simulink model "carSim"  (R2020a)
settings: Solver=FixedStepAuto  StartTime=0.0  StopTime=150  FixedStep=0.1406  MaxStep=0.1  RelTol=1e-3
model workspace: external: MATLAB File C:\Users\chsl\Documents\teaching\Reguleringsteknik (4. semester)\matlab\handInExercises\ex2Init.m (data not in the file)
values from neighbouring files (symbols this model uses):
  c = 10    [ex2Init.m]
  g = 9.82    [ex2Init.m]
  m = 900    [ex2Init.m]
  vBar = 10    [ex2Init.m]
settings Model: Creator=chsl  LastModifiedBy=madsw
settings DataIOCC: ReturnWorkspaceOutputs=off
settings DebuggingCC: ArithmeticOperatorsInVariantConditions=warning
settings SFSimCC: SimUseLocalCustomCode=off  CustomCodeUndefinedFunction=UseInterfaceOnly
settings RTWCC: RTWUseLocalCustomCode=off

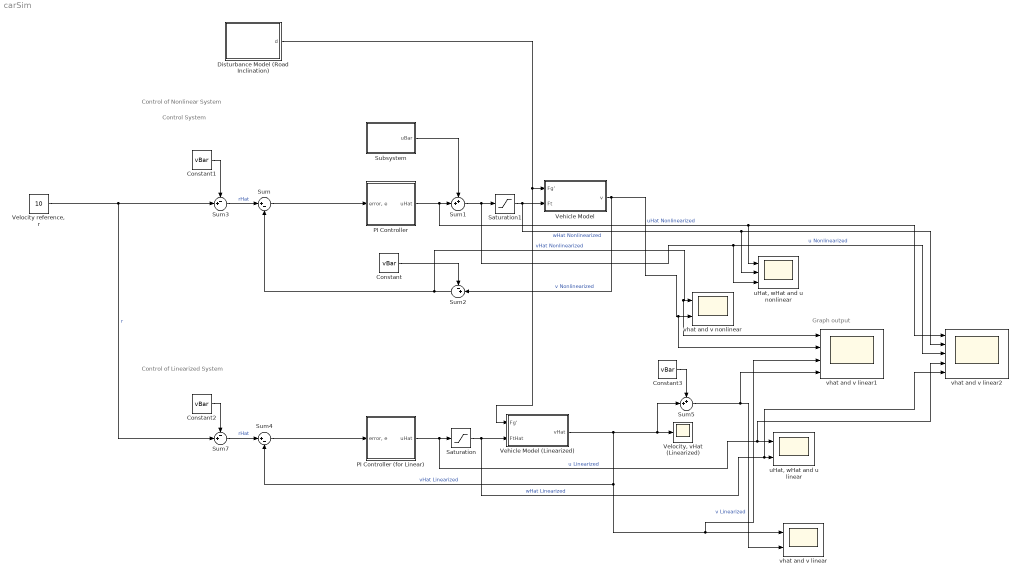
== system carSim ==
  note: Graph output
  note: Control System
  note: Control of Nonlinear System
  note: Control of Linearized System
  Constant{,1..3} (4 alike) : Constant  Value=vBar
  "Disturbance Model (Road Inclination) " : Subsystem
  PI Controller : Subsystem
  PI Controller (for Linear) : Subsystem
  Saturation : Saturate  UpperLimit=3000  LowerLimit=-3000
  Saturation1 : Saturate  UpperLimit=3000  LowerLimit=-3000
  Subsystem : Subsystem
  Sum : Sum  Inputs=|+-
  Sum1 : Sum  Inputs=++|
  Sum2 : Sum  Inputs=-+|
  Sum3 : Sum  Inputs=-+|
  Sum4 : Sum  Inputs=|+-
  Sum5 : Sum  Inputs=++|
  Sum7 : Sum  Inputs=-+|
  Vehicle Model : Subsystem
  Vehicle Model (Linearized) : Subsystem
  "Velocity reference, r" : Constant  Value=10
  "Velocity, vHat (Linearized)" : Scope
  "uHat, wHat and u linear" : Scope  NumInputPorts=2
  "uHat, wHat and u nonlinear" : Scope  NumInputPorts=3
  vhat and v linear : Scope  NumInputPorts=2
  vhat and v linear1 : Scope  NumInputPorts=4
  vhat and v linear2 : Scope  NumInputPorts=5
  vhat and v nonlinear : Scope  NumInputPorts=2
  wires:
  "Disturbance Model (Road Inclination) "/1(d) -> Vehicle Model (Linearized)/1(Fg'), Vehicle Model/1(Fg')
  Sum/1 -> PI Controller/1("error, e")
  Sum1/1 -> Saturation1/1, vhat and v linear2/3, "uHat, wHat and u nonlinear"/3  "u Nonlinearized"
  PI Controller/1(uHat) -> "uHat, wHat and u nonlinear"/1, vhat and v linear2/1, Sum1/2  "uHat Nonlinearized"
  Subsystem/1(uBar) -> Sum1/1
  Constant/1 -> Sum2/1
  Vehicle Model/1(v) -> Sum2/2, vhat and v linear1/2, vhat and v nonlinear/2  "v Nonlinearized"
  Sum2/1 -> vhat and v linear1/1, vhat and v nonlinear/1, Sum/2  "vHat Nonlinearized"
  Constant1/1 -> Sum3/1
  Sum4/1 -> PI Controller (for Linear)/1("error, e")
  Sum3/1 -> Sum/1  "rHat"
  PI Controller (for Linear)/1(uHat) -> vhat and v linear2/4, "uHat, wHat and u linear"/1, Saturation/1  "u Linearized"
  Constant2/1 -> Sum7/1
  "Velocity reference, r"/1 -> Sum7/2, Sum3/2  "r"
  Sum7/1 -> Sum4/1  "rHat"
  Constant3/1 -> Sum5/1
  Sum5/1 -> vhat and v linear/2, vhat and v linear1/4  "v Linearized"
  Saturation1/1 -> Vehicle Model/2(Ft), vhat and v linear2/2, "uHat, wHat and u nonlinear"/2  "wHat Nonlinearized"
  Vehicle Model (Linearized)/1(vHat) -> vhat and v linear1/3, vhat and v linear/1, Sum4/2, Sum5/2, "Velocity, vHat (Linearized)"/1  "vHat Linearized"
  Saturation/1 -> vhat and v linear2/5, "uHat, wHat and u linear"/2, Vehicle Model (Linearized)/2(FtHat)  "wHat Linearized"

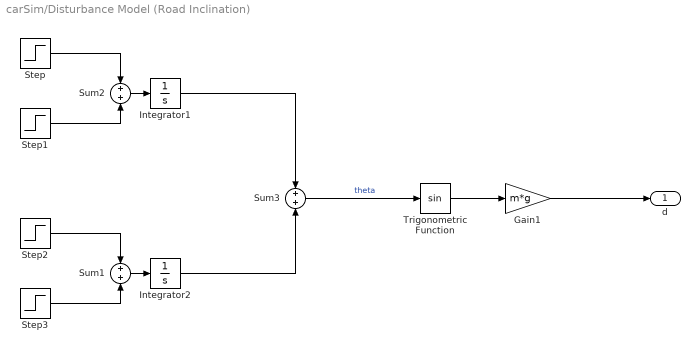
== system carSim/Disturbance Model (Road Inclination)  ==
  Gain1 : Gain  Gain=m*g
  Integrator1 : Integrator
  Integrator2 : Integrator
  Step : Step  Time=50  After=0.01  SampleTime=0
  Step1 : Step  Time=60  After=-0.01  SampleTime=0
  Step2 : Step  Time=100  After=0.1  SampleTime=0
  Step3 : Step  Time=110  After=-0.1  SampleTime=0
  Sum1 : Sum
  Sum2 : Sum
  Sum3 : Sum
  Trigonometric Function : Trigonometry
  d : Outport  VectorParamsAs1DForOutWhenUnconnected=off
  wires:
  Step/1 -> Sum2/1
  Sum2/1 -> Integrator1/1
  Step1/1 -> Sum2/2
  Integrator1/1 -> Sum3/1
  Sum1/1 -> Integrator2/1
  Step3/1 -> Sum1/2
  Step2/1 -> Sum1/1
  Integrator2/1 -> Sum3/2
  Trigonometric Function/1 -> Gain1/1
  Sum3/1 -> Trigonometric Function/1  "theta"
  Gain1/1 -> d/1

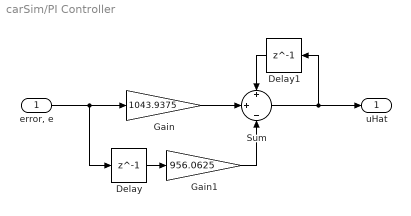
== system carSim/PI Controller ==
  "error, e" : Inport
  Delay : Delay  DelayLength=1
  Delay1 : Delay  DelayLength=1
  Gain : Gain  Gain=1043.9375
  Gain1 : Gain  Gain=956.0625
  Sum : Sum  Inputs=+|+|-
  uHat : Outport  VectorParamsAs1DForOutWhenUnconnected=off
  wires:
  "error, e"/1 -> Delay/1, Gain/1
  Delay/1 -> Gain1/1
  Gain/1 -> Sum/2
  Gain1/1 -> Sum/3
  Sum/1 -> uHat/1, Delay1/1
  Delay1/1 -> Sum/1

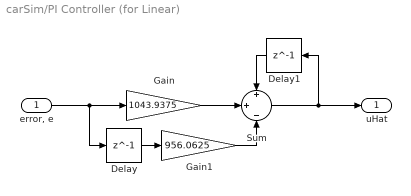
== system carSim/PI Controller (for Linear) ==
  "error, e" : Inport
  Delay : Delay  DelayLength=1
  Delay1 : Delay  DelayLength=1
  Gain : Gain  Gain=1043.9375
  Gain1 : Gain  Gain=956.0625
  Sum : Sum  Inputs=+|+|-
  uHat : Outport  VectorParamsAs1DForOutWhenUnconnected=off
  wires:
  "error, e"/1 -> Delay/1, Gain/1
  Delay/1 -> Gain1/1
  Gain/1 -> Sum/2
  Gain1/1 -> Sum/3
  Sum/1 -> uHat/1, Delay1/1
  Delay1/1 -> Sum/1

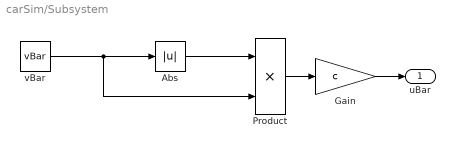
== system carSim/Subsystem ==
  Abs : Abs
  Gain : Gain  Gain=c
  Product : Product
  vBar : Constant  Value=vBar
  uBar : Outport  VectorParamsAs1DForOutWhenUnconnected=off
  wires:
  vBar/1 -> Product/2, Abs/1
  Gain/1 -> uBar/1
  Abs/1 -> Product/1
  Product/1 -> Gain/1

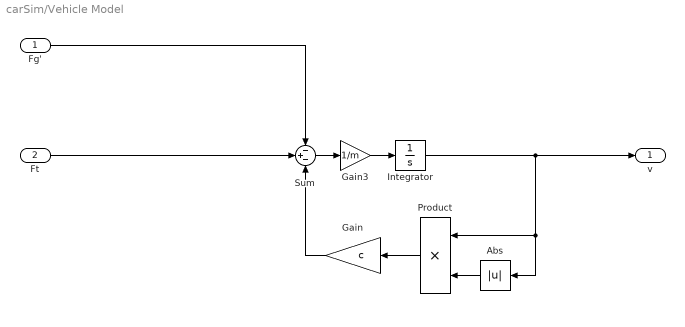
== system carSim/Vehicle Model ==
  Fg' : Inport
  Ft : Inport  Port=2
  Abs : Abs
  Gain : Gain  Gain=c
  Gain3 : Gain  Gain=1/m
  Integrator : Integrator  InitialCondition=vBar
  Product : Product
  Sum : Sum  Inputs=-+-
  v : Outport  VectorParamsAs1DForOutWhenUnconnected=off
  wires:
  Fg'/1 -> Sum/1
  Integrator/1 -> Abs/1, Product/1, v/1
  Sum/1 -> Gain3/1
  Gain3/1 -> Integrator/1
  Gain/1 -> Sum/3
  Abs/1 -> Product/2
  Product/1 -> Gain/1
  Ft/1 -> Sum/2

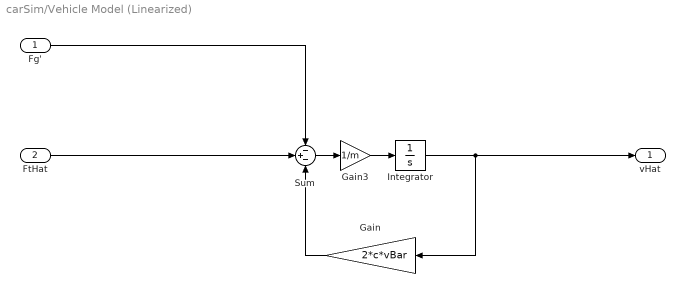
== system carSim/Vehicle Model (Linearized) ==
  Fg' : Inport
  FtHat : Inport  Port=2
  Gain : Gain  Gain=2*c*vBar
  Gain3 : Gain  Gain=1/m
  Integrator : Integrator
  Sum : Sum  Inputs=-+-
  vHat : Outport  VectorParamsAs1DForOutWhenUnconnected=off
  wires:
  Sum/1 -> Gain3/1
  FtHat/1 -> Sum/2
  Gain3/1 -> Integrator/1
  Gain/1 -> Sum/3
  Integrator/1 -> Gain/1, vHat/1
  Fg'/1 -> Sum/1
